simulink model "Direct_Form_realiz"  (R2020a)
settings: Solver=VariableStepAuto  StartTime=0.0  StopTime=10.0  RelTol=1e-3
settings Model: Creator=DELL  LastModifiedBy=DELL

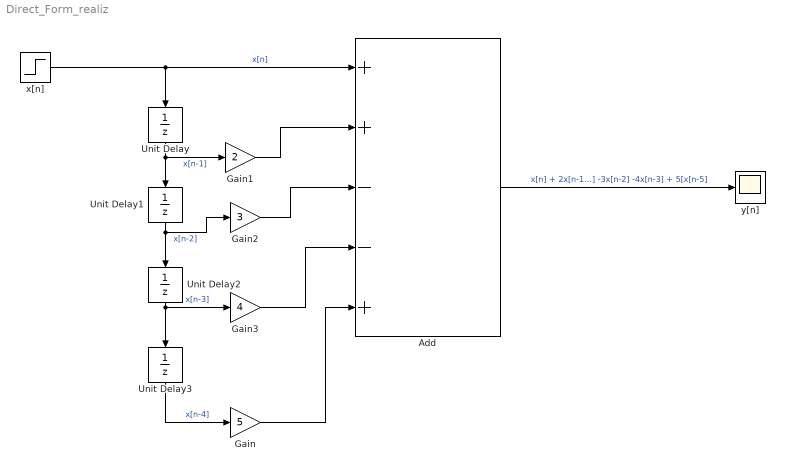
== system Direct_Form_realiz ==
  Add : Sum  Inputs=++--+
  Gain : Gain  Gain=5
  Gain1 : Gain  Gain=2
  Gain2 : Gain  Gain=3
  Gain3 : Gain  Gain=4
  Unit Delay{,1..3} (4 alike) : UnitDelay  SampleTime=-1  HasFrameUpgradeWarning=on
  x[n] : Step  SampleTime=0
  y[n] : Scope
  wires:
  x[n]/1 -> Unit Delay/1, Add/1  "x[n]"
  Unit Delay/1 -> Gain1/1, Unit Delay1/1  "x[n-1]"
  Unit Delay1/1 -> Gain2/1, Unit Delay2/1  "x[n-2]"
  Unit Delay2/1 -> Unit Delay3/1, Gain3/1  "x[n-3]"
  Unit Delay3/1 -> Gain/1  "x[n-4]"
  Gain1/1 -> Add/2
  Gain2/1 -> Add/3
  Gain3/1 -> Add/4
  Gain/1 -> Add/5
  Add/1 -> y[n]/1  "x[n] + 2x[n-1] -3x[n-2] -4x[n-3] + 5[x[n-5]"
